simulink model "OsCar_Simulink_Model"  (R2024a)
settings: Solver=VariableStepAuto  StartTime=0.0  StopTime=11  RelTol=1e-3
libraries: shared6dof x1
settings Model: Creator=ahssa  LastModifiedBy=Ahssan
settings RTWCC: GPUComputeCapability=3.5

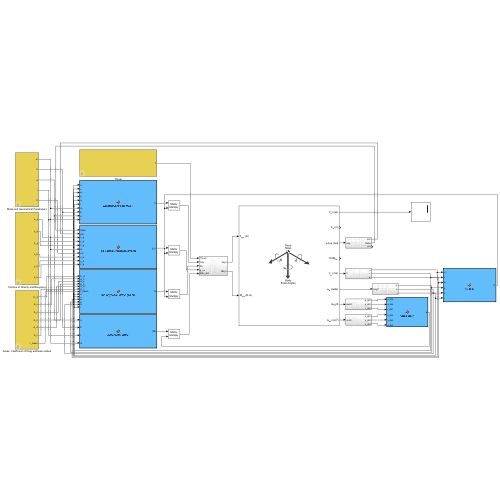
[thumbnail: Simulink's stored preview of the top-level diagram]
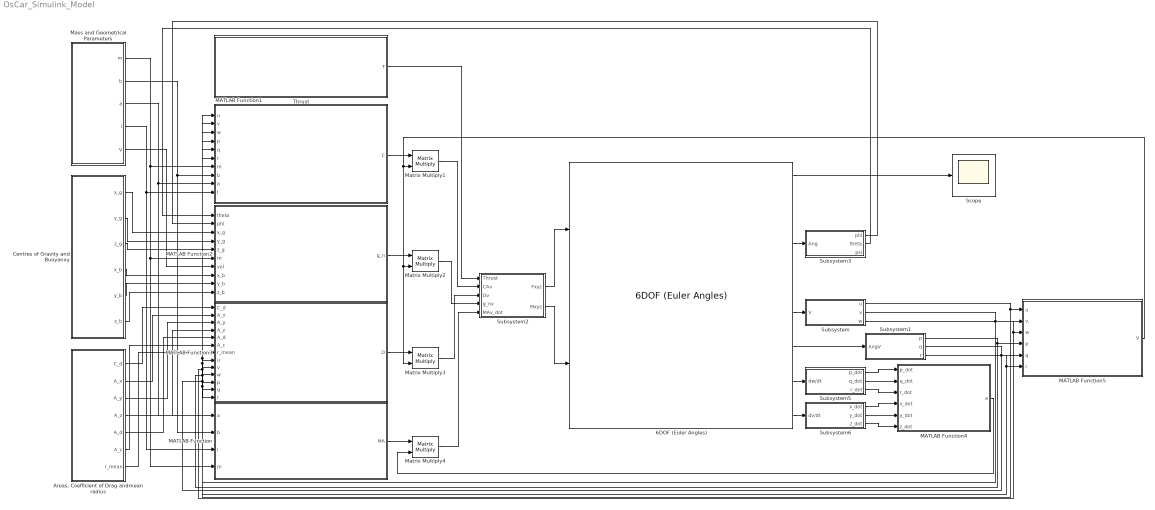
== system OsCar_Simulink_Model ==
  6DOF (Euler Angles) : shared6dof/6DOF (Euler Angles)  units=Metric (MKS)  mtype=Fixed  rep=Euler Angles  xme_0=[0 0 0]  Vm_0=[0 0 0]  eul_0=[0 0 0]  pm_0=[0 0 0]  mass_0=2.8777  mass_e=0.5  mass_f=2.0  inertia=[0.004251,0,0;0,0.028969,0;0,0,0.028969]  inertia_e=eye(3)  inertia_f=2*eye(3)  k_quat=1.0  vre_flag=on  abi_flag=off  aMode=0  xme_statename=''  Vm_statename=''  eul_statename=''  quat_statename=''  pm_statename=''  mass_statename=''
  "Areas, Coefficient of Drag andmean radius" : Subsystem
      mask DialogControl Control2 Prompt: (Add text here)
  Centres of Gravity and Buoyanxy : Subsystem
      mask DialogControl Control2 Prompt: Centres of gravity and buoyancy
  MATLAB Function : MATLAB Function  TreatAsAtomicUnit=on
  MATLAB Function1 : MATLAB Function  TreatAsAtomicUnit=on
  MATLAB Function2 : MATLAB Function  TreatAsAtomicUnit=on
  MATLAB Function3 : MATLAB Function  TreatAsAtomicUnit=on
  MATLAB Function4 : MATLAB Function  TreatAsAtomicUnit=on
  MATLAB Function5 : MATLAB Function  TreatAsAtomicUnit=on
  Mass and Geometrical Parameters : Subsystem
      mask DialogControl Control2 Prompt: Mass and Geometrical Parameters
  Matrix Multiply{1..4} (4 alike) : Product  Multiplication=Matrix(*)
  Scope : Scope
  Subsystem : Subsystem
  Subsystem1 : Subsystem
  Subsystem2 : Subsystem
  Subsystem3 : Subsystem
  Subsystem5 : Subsystem
  Subsystem6 : Subsystem
  Thrust : Subsystem
      mask DialogControl Control2 Prompt: Thrust
  wires:
  6DOF (Euler Angles)/5 -> Subsystem/1(V)
  Subsystem/1(u) -> MATLAB Function5/1(u), MATLAB Function1/1(u), MATLAB Function3/8(u)
  Subsystem/2(v) -> MATLAB Function1/2(v), MATLAB Function3/9(v), MATLAB Function5/2(v)
  Subsystem/3(w) -> MATLAB Function1/3(w), MATLAB Function3/10(w), MATLAB Function5/3(w)
  6DOF (Euler Angles)/6 -> Subsystem1/1(AngV)
  Subsystem1/1(p) -> MATLAB Function5/4(p), MATLAB Function1/4(p), MATLAB Function3/11(p)
  Subsystem1/2(q) -> MATLAB Function5/5(q), MATLAB Function1/5(q), MATLAB Function3/12(q)
  Subsystem1/3(r) -> MATLAB Function5/6(r), MATLAB Function1/6(r), MATLAB Function3/13(r)
  MATLAB Function1/1(C) -> Matrix Multiply1/1
  MATLAB Function2/1(g_n) -> Matrix Multiply2/1
  MATLAB Function3/1(D) -> Matrix Multiply3/1
  MATLAB Function5/1(V) -> Matrix Multiply3/2, Matrix Multiply2/2, Matrix Multiply1/2
  Thrust/1(T) -> Subsystem2/1(Thrust)
  Matrix Multiply1/1 -> Subsystem2/2(CAv)
  Matrix Multiply2/1 -> Subsystem2/4(g_nv)
  Matrix Multiply3/1 -> Subsystem2/3(Dv)
  Subsystem2/1(Fxyz) -> 6DOF (Euler Angles)/1
  Subsystem2/2(Mxyz) -> 6DOF (Euler Angles)/2
  6DOF (Euler Angles)/3 -> Subsystem3/1(Ang)
  Subsystem3/1(phi) -> MATLAB Function2/2(phi)
  Subsystem3/2(theta) -> MATLAB Function2/1(theta)
  6DOF (Euler Angles)/1 -> Scope/1
  MATLAB Function/1(MA) -> Matrix Multiply4/1
  Matrix Multiply4/1 -> Subsystem2/5(MAv_dot)
  6DOF (Euler Angles)/8 -> Subsystem6/1(dv/dt)
  6DOF (Euler Angles)/7 -> Subsystem5/1(dw/dt)
  Subsystem6/2(y_dot) -> MATLAB Function4/5(y_dot)
  Subsystem6/3(z_dot) -> MATLAB Function4/6(z_dot)
  Subsystem6/1(x_dot) -> MATLAB Function4/4(x_dot)
  Subsystem5/3(r_dot) -> MATLAB Function4/3(r_dot)
  Subsystem5/2(q_dot) -> MATLAB Function4/2(q_dot)
  Subsystem5/1(p_dot) -> MATLAB Function4/1(p_dot)
  MATLAB Function4/1(a) -> Matrix Multiply4/2
  Centres of Gravity and Buoyanxy/4(x_b) -> MATLAB Function2/8(x_b)
  Centres of Gravity and Buoyanxy/5(y_b) -> MATLAB Function2/9(y_b)
  Centres of Gravity and Buoyanxy/6(z_b) -> MATLAB Function2/10(z_b)
  Centres of Gravity and Buoyanxy/1(x_g) -> MATLAB Function2/3(x_g)
  Centres of Gravity and Buoyanxy/2(y_g) -> MATLAB Function2/4(y_g)
  Centres of Gravity and Buoyanxy/3(z_g) -> MATLAB Function2/5(z_g)
  "Areas, Coefficient of Drag andmean radius"/1(C_d) -> MATLAB Function3/1(C_d)
  "Areas, Coefficient of Drag andmean radius"/2(A_x) -> MATLAB Function3/2(A_x)
  "Areas, Coefficient of Drag andmean radius"/3(A_y) -> MATLAB Function3/3(A_y)
  "Areas, Coefficient of Drag andmean radius"/4(A_z) -> MATLAB Function3/4(A_z)
  "Areas, Coefficient of Drag andmean radius"/5(A_d) -> MATLAB Function3/5(A_d)
  "Areas, Coefficient of Drag andmean radius"/6(A_c) -> MATLAB Function3/6(A_c)
  "Areas, Coefficient of Drag andmean radius"/7(r_mean) -> MATLAB Function3/7(r_mean)
  Mass and Geometrical Parameters/3(a) -> MATLAB Function1/9(a), MATLAB Function/1(a)
  Mass and Geometrical Parameters/1(m) -> MATLAB Function/4(m), MATLAB Function2/6(m), MATLAB Function1/7(m)
  Mass and Geometrical Parameters/4(l) -> MATLAB Function/3(l), MATLAB Function1/10(l)
  Mass and Geometrical Parameters/2(b) -> MATLAB Function1/8(b), MATLAB Function/2(b)
  Mass and Geometrical Parameters/5(V) -> MATLAB Function2/7(vol)

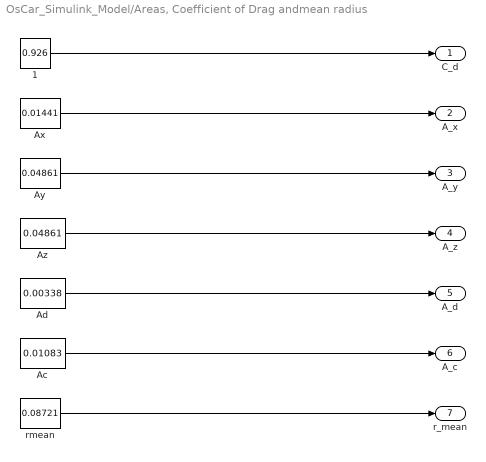
== system OsCar_Simulink_Model/Areas, Coefficient of Drag andmean radius ==
  1 : Constant  Value=0.926
  Ac : Constant  Value=0.01083
  Ad : Constant  Value=0.00338
  Ax : Constant  Value=0.01441
  Ay : Constant  Value=0.04861
  Az : Constant  Value=0.04861
  rmean : Constant  Value=0.08721
  C_d : Outport
  A_x : Outport  Port=2
  A_y : Outport  Port=3
  A_z : Outport  Port=4
  A_d : Outport  Port=5
  A_c : Outport  Port=6
  r_mean : Outport  Port=7
  wires:
  Ax/1 -> A_x/1
  rmean/1 -> r_mean/1
  Ac/1 -> A_c/1
  Az/1 -> A_z/1
  Ay/1 -> A_y/1
  Ad/1 -> A_d/1
  1/1 -> C_d/1

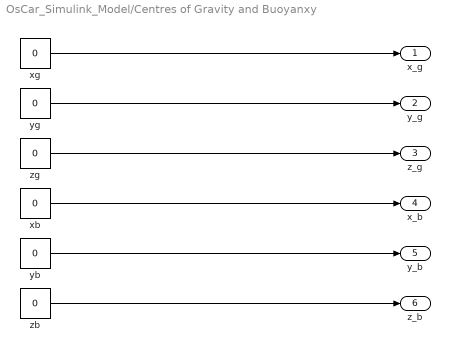
== system OsCar_Simulink_Model/Centres of Gravity and Buoyanxy ==
  xb : Constant  Value=0
  xg : Constant  Value=0
  yb : Constant  Value=0
  yg : Constant  Value=0
  zb : Constant  Value=0
  zg : Constant  Value=0
  x_g : Outport
  y_g : Outport  Port=2
  z_g : Outport  Port=3
  x_b : Outport  Port=4
  y_b : Outport  Port=5
  z_b : Outport  Port=6
  wires:
  xg/1 -> x_g/1
  yg/1 -> y_g/1
  zg/1 -> z_g/1
  yb/1 -> y_b/1
  xb/1 -> x_b/1
  zb/1 -> z_b/1

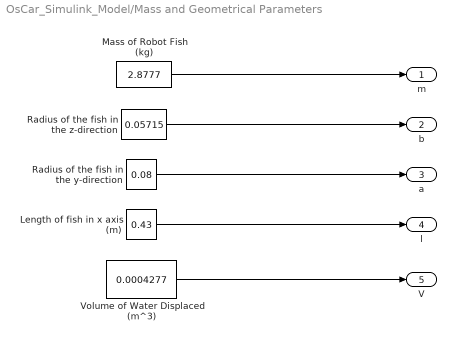
== system OsCar_Simulink_Model/Mass and Geometrical Parameters ==
  Length of fish in x axis (m) : Constant  Value=0.43
  Mass of Robot Fish (kg) : Constant  Value=2.8777
  Radius of the fish in the y-direction : Constant  Value=0.08
  Radius of the fish in the z-direction : Constant  Value=0.05715
  Volume of Water Displaced (m^3) : Constant  Value=0.0004277
  m : Outport
  b : Outport  Port=2
  a : Outport  Port=3
  l : Outport  Port=4
  V : Outport  Port=5
  wires:
  Radius of the fish in the y-direction/1 -> a/1
  Mass of Robot Fish (kg)/1 -> m/1
  Length of fish in x axis (m)/1 -> l/1
  Radius of the fish in the z-direction/1 -> b/1
  Volume of Water Displaced (m^3)/1 -> V/1

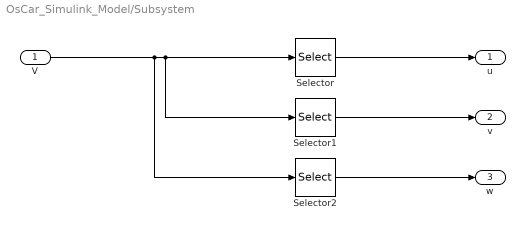
== system OsCar_Simulink_Model/Subsystem ==
  V : Inport
  Selector : Selector  InputPortWidth=3  IndexOptions=Index vector (dialog)  Indices=[1]  OutputSizes=1
  Selector1 : Selector  InputPortWidth=3  IndexOptions=Index vector (dialog)  Indices=[2]  OutputSizes=1
  Selector2 : Selector  InputPortWidth=3  IndexOptions=Index vector (dialog)  Indices=[2]  OutputSizes=1
  u : Outport
  v : Outport  Port=2
  w : Outport  Port=3
  wires:
  V/1 -> Selector2/1, Selector1/1, Selector/1
  Selector/1 -> u/1
  Selector1/1 -> v/1
  Selector2/1 -> w/1

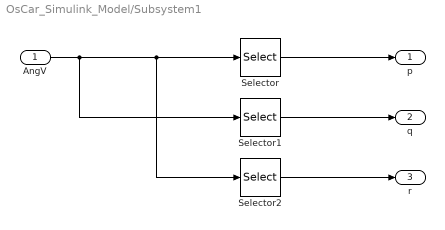
== system OsCar_Simulink_Model/Subsystem1 ==
  AngV : Inport
  Selector : Selector  InputPortWidth=3  IndexOptions=Index vector (dialog)  Indices=[1]  OutputSizes=1
  Selector1 : Selector  InputPortWidth=3  IndexOptions=Index vector (dialog)  Indices=[2]  OutputSizes=1
  Selector2 : Selector  InputPortWidth=3  IndexOptions=Index vector (dialog)  Indices=[3]  OutputSizes=1
  p : Outport
  q : Outport  Port=2
  r : Outport  Port=3
  wires:
  AngV/1 -> Selector1/1, Selector2/1, Selector/1
  Selector/1 -> p/1
  Selector1/1 -> q/1
  Selector2/1 -> r/1

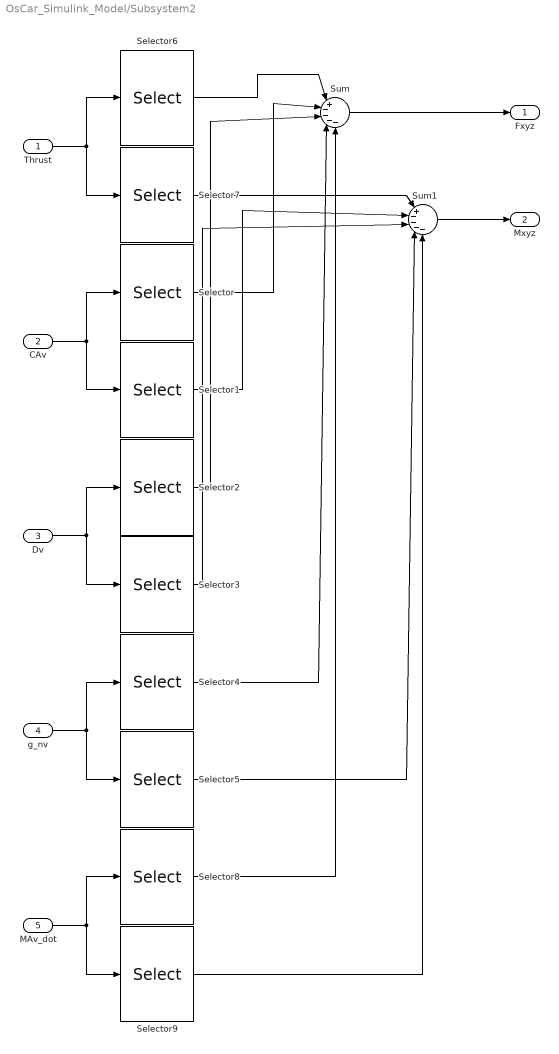
== system OsCar_Simulink_Model/Subsystem2 ==
  Thrust : Inport
  CAv : Inport  Port=2
  Dv : Inport  Port=3
  g_nv : Inport  Port=4
  MAv_dot : Inport  Port=5
  Selector{,2,4,6,8} (5 alike) : Selector  InputPortWidth=6  IndexOptions=Index vector (dialog)  Indices=[1 2 3]  OutputSizes=1
  Selector{1,3,5,7,9} (5 alike) : Selector  InputPortWidth=6  IndexOptions=Index vector (dialog)  Indices=[4 5 6]  OutputSizes=1
  Sum : Sum  Inputs=|+----
  Sum1 : Sum  Inputs=|+----
  Fxyz : Outport
  Mxyz : Outport  Port=2
  wires:
  CAv/1 -> Selector1/1, Selector/1
  Dv/1 -> Selector3/1, Selector2/1
  g_nv/1 -> Selector4/1, Selector5/1
  Thrust/1 -> Selector6/1, Selector7/1
  Selector6/1 -> Sum/1
  Selector/1 -> Sum/2
  Selector2/1 -> Sum/3
  Selector4/1 -> Sum/4
  Sum/1 -> Fxyz/1
  Selector7/1 -> Sum1/1
  Selector1/1 -> Sum1/2
  Selector3/1 -> Sum1/3
  Selector5/1 -> Sum1/4
  Sum1/1 -> Mxyz/1
  MAv_dot/1 -> Selector9/1, Selector8/1
  Selector8/1 -> Sum/5
  Selector9/1 -> Sum1/5

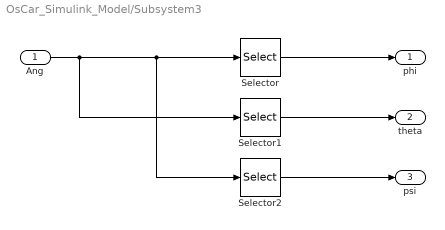
== system OsCar_Simulink_Model/Subsystem3 ==
  Ang : Inport
  Selector : Selector  InputPortWidth=3  IndexOptions=Index vector (dialog)  Indices=[1]  OutputSizes=1
  Selector1 : Selector  InputPortWidth=3  IndexOptions=Index vector (dialog)  Indices=[2]  OutputSizes=1
  Selector2 : Selector  InputPortWidth=3  IndexOptions=Index vector (dialog)  Indices=[3]  OutputSizes=1
  phi : Outport
  theta : Outport  Port=2
  psi : Outport  Port=3
  wires:
  Ang/1 -> Selector1/1, Selector2/1, Selector/1
  Selector/1 -> phi/1
  Selector1/1 -> theta/1
  Selector2/1 -> psi/1

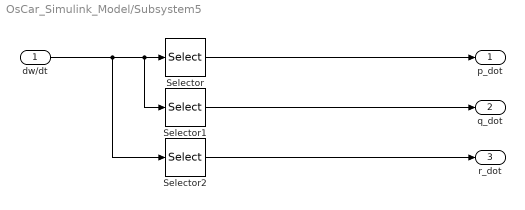
== system OsCar_Simulink_Model/Subsystem5 ==
  dw/dt : Inport
  Selector : Selector  InputPortWidth=3  IndexOptions=Index vector (dialog)  Indices=[1]  OutputSizes=1
  Selector1 : Selector  InputPortWidth=3  IndexOptions=Index vector (dialog)  Indices=[2]  OutputSizes=1
  Selector2 : Selector  InputPortWidth=3  IndexOptions=Index vector (dialog)  Indices=[3]  OutputSizes=1
  p_dot : Outport
  q_dot : Outport  Port=2
  r_dot : Outport  Port=3
  wires:
  dw/dt/1 -> Selector2/1, Selector1/1, Selector/1
  Selector/1 -> p_dot/1
  Selector1/1 -> q_dot/1
  Selector2/1 -> r_dot/1

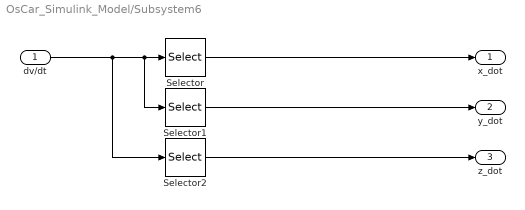
== system OsCar_Simulink_Model/Subsystem6 ==
  dv/dt : Inport
  Selector : Selector  InputPortWidth=3  IndexOptions=Index vector (dialog)  Indices=[1]  OutputSizes=1
  Selector1 : Selector  InputPortWidth=3  IndexOptions=Index vector (dialog)  Indices=[2]  OutputSizes=1
  Selector2 : Selector  InputPortWidth=3  IndexOptions=Index vector (dialog)  Indices=[3]  OutputSizes=1
  x_dot : Outport
  y_dot : Outport  Port=2
  z_dot : Outport  Port=3
  wires:
  dv/dt/1 -> Selector2/1, Selector1/1, Selector/1
  Selector/1 -> x_dot/1
  Selector1/1 -> y_dot/1
  Selector2/1 -> z_dot/1

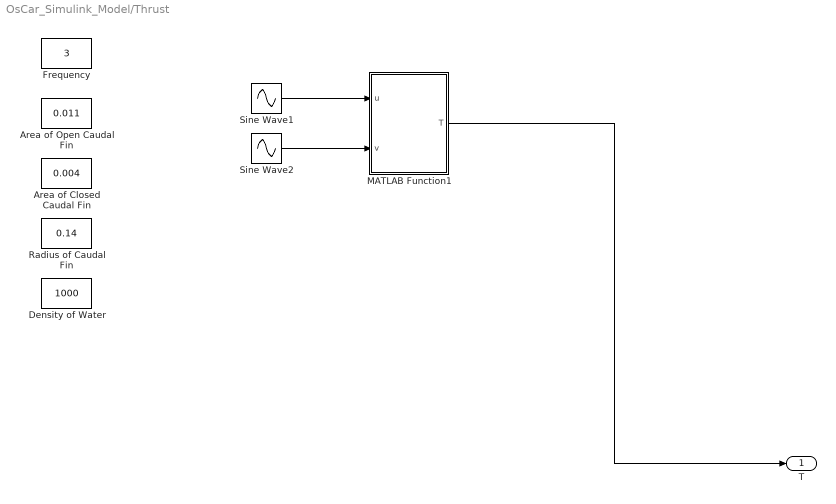
== system OsCar_Simulink_Model/Thrust ==
  Area of Closed Caudal Fin : Constant  Value=0.004
  Area of Open Caudal Fin : Constant  Value=0.011
  Density of Water : Constant  Value=1000
  Frequency : Constant  Value=3
  MATLAB Function1 : MATLAB Function  TreatAsAtomicUnit=on
  Radius of Caudal Fin : Constant  Value=0.14
  Sine Wave1 : Sin  Amplitude=7/36*pi  Frequency=2*pi*3  SampleTime=0
  Sine Wave2 : Sin  Amplitude=sqrt(1/2* 1000 * 0.011 * 0.14^2 * (7/36*pi)^2 * 4*pi^2 * (3)^2)  Frequency=2*pi*3  Phase=pi/2  SampleTime=0
  T : Outport
  wires:
  Sine Wave1/1 -> MATLAB Function1/1(u)
  Sine Wave2/1 -> MATLAB Function1/2(v)
  MATLAB Function1/1(T) -> T/1

== matlab function OsCar_Simulink_Model/Thrust/MATLAB Function1 ==
  data: u input; T output; v input
function T = fcn(u,v)
A = (cos(u))^2;
B = (v)^2;
T_x = A*B;
T = [T_x;
    0;
    0;
    0;
    0;
    0];
end

== matlab function OsCar_Simulink_Model/MATLAB Function1 ==
  data: u input; v input; w input; p input; q input; r input; m input; b input; a input; C output; l input
function C = CoriolisisCentripetalMatrix(u,v,w,p,q,r,m,b,a,l)
c = l/2;
vol = 4/3*pi*a*b*c;
I_yy = 1/5*m*(a^2+c^2);
I_zz = 1/5*m*(a^2+c^2);
e = sqrt(1-(b/a)^2);
alpha_0 = 2*(1-e^2)/e^3 *(1/2*log((1+e)/(1-e))-e);
beta_0 = 1/e^2 - (1-e^2)/(2*e^3) * log((1+e)/(1-e));
k1 = alpha_0 / (2-alpha_0);
k2 = beta_0 / (2-beta_0);
k_prime = e^4*(beta_0 - alpha_0)/((2-e^2) * (2*e^2-(2-e^2)*(beta_0 - alpha_0)));
X_u_dot = k1 * m;
Y_v_dot = k2 * m;
Z_w_dot = k2 * m;
K_p_dot = 0;
M_q_dot = k_prime * I_yy;
N_r_dot = k_prime * I_zz;
% CRB = [0, 0, 0, m*z_g*r, m*w, -m*v;
%     0, 0, 0, -m*w, m*z_g*r, m*u;
%     0, 0, 0, -m*alpha_1, -m*alpha_2, 0;
%     -m*z_g*r, m*w, m*alpha_1, 0, Izz*r, -Iyy*q;
%     -m*w, -m*z_g*r, m*alpha_2, -Izz*r, 0, Ixx*p;
%     m*v, -m*u, 0, Iyy*q, -Ixx*p, 0];
CA = [0, 0, 0, 0, -Z_w_dot*w, Y_v_dot*v;
    0, 0, 0, Z_w_dot*w, 0, -X_u_dot*u;
    0, 0, 0, -Y_v_dot*v, X_u_dot*u, 0;
    0, -Z_w_dot*w, Y_v_dot*v, 0, -N_r_dot*r, M_q_dot*q;
    Z_w_dot*w, 0, -X_u_dot*u, N_r_dot*r, 0, -K_p_dot*p;
    -Y_v_dot*v, X_u_dot*u, 0, -M_q_dot*q, K_p_dot*p, 0];
C = CA;
end

== matlab function OsCar_Simulink_Model/MATLAB Function2 ==
  data: theta input; phi input; x_g input; y_g input; z_g input; m input; vol input; x_b input; y_b input; z_b input; g_n output
function g_n = HydrostaticForcesandMoments(theta,phi,x_g,y_g,z_g,m,vol,x_b,y_b,z_b)
w = m*9.814;
b = 1000*9.814*vol;
g_n = [(w-b)*sin(theta), 0, 0, 0, 0, 0; 
    0, -(w-b)*cos(theta)*sin(phi), 0, 0, 0, 0;
    0, 0, -(w-b)*cos(phi)*sin(theta), 0, 0, 0;
    0, 0, 0, -(y_g*w-y_b*b)*cos(theta)*cos(phi)+(z_g*w-z_b*b)*cos(theta)*sin(phi), 0, 0;
    0, 0, 0, 0, (x_g*w-x_b*b)*cos(theta)*cos(phi)+(z_g*w-z_b*b)*sin(theta), 0;
    0, 0, 0, 0, 0, (x_g*w-x_b*b)*cos(theta)*sin(phi)-(y_g*w-y_b*b)*sin(theta)];
end

== matlab function OsCar_Simulink_Model/MATLAB Function3 ==
  data: C_d input; A_x input; A_y input; A_z input; A_d input; A_c input; r_mean input; u input; v input; w input; D output; p input; q input; r input
function D = HydrodynamicDampingMatrix(C_d,A_x,A_y,A_z,A_d, A_c,r_mean,u,v,w,p,q,r)
t = 1;
C_d_f = 0.1 + 0.7*t;
rho_w = 1000;
X_u_u = -1/2*rho_w*C_d*A_x;
Y_v_v = -1/2*rho_w*C_d*A_y - 1/2*rho_w*A_d*C_d_f - 1/2*rho_w*A_c*C_d_f;
Z_w_w = -1/2*rho_w*C_d*A_z;
K_p_p = Y_v_v*(r_mean)^3;
M_q_q = Z_w_w*(r_mean)^3;
N_r_r = X_u_u*(r_mean)^3;
X_u = -31;
Y_v = 0;
Z_w = 0;
K_p = 0;
M_q = 0;
N_r = 0;
D = -diag([X_u,Y_v,Z_w,K_p,M_q,N_r]) - diag([X_u_u*abs(u), Y_v_v*abs(v), Z_w_w*abs(w), K_p_p*abs(p), M_q_q*abs(q), N_r_r*abs(r)]);
end

== matlab function OsCar_Simulink_Model/MATLAB Function ==
  data: a input; MA output; b input; l input; m input
function MA = AddedMassMatrix(a,b,l,m)
c = l/2;
m = 2.877;
vol = 4/3*pi*a*b*c;
I_yy = 1/5*m*(a^2+c^2);
I_zz = 1/5*m*(a^2+c^2);
e = sqrt(1-(b/a)^2);
alpha_0 = 2*(1-e^2)/e^3 *(1/2*log((1+e)/(1-e))-e);
beta_0 = 1/e^2 - (1-e^2)/(2*e^3) * log((1+e)/(1-e));
k1 = alpha_0 / (2-alpha_0);
k2 = beta_0 / (2-beta_0);
k_prime = e^4*(beta_0 - alpha_0)/((2-e^2) * (2*e^2-(2-e^2)*(beta_0 - alpha_0)));
X_u_dot = k1 * m;
Y_v_dot = k2 * m;
Z_w_dot = k2 * m;
K_p_dot = 0;
M_q_dot = k_prime * I_yy;
N_r_dot = k_prime * I_zz;
MA = diag([X_u_dot, Y_v_dot, Z_w_dot, K_p_dot, M_q_dot, N_r_dot]);
end

== matlab function OsCar_Simulink_Model/MATLAB Function5 ==
  data: u input; V output; v input; w input; p input; q input; r input
function V  = Velocity(u,v,w,p,q,r)
V = [u;v;w;p;q;r];
end

== matlab function OsCar_Simulink_Model/MATLAB Function4 ==
  data: p_dot input; q_dot input; r_dot input; x_dot input; a output; y_dot input; z_dot input
function a = Acceleration(p_dot,q_dot,r_dot,x_dot,y_dot,z_dot)
a = [x_dot;
    y_dot;
    z_dot;
    p_dot;
    q_dot;
    r_dot];
end
